simulink model "Tracker_with_Position_Control"  (R2024b)
settings: Solver=FixedStepDiscrete  StartTime=0.0  StopTime=inf  FixedStep=0.005  RelTol=1e-3  EnableMultiTasking=on
libraries: arduinolib x3, simulink x1, arduinosensorlib x1, simulink_extras x1, slpidlib x1
settings Model: ExtModeTrigDuration=2  Creator=yoany  LastModifiedBy=shaha
settings OptimizationCC: DefaultUnderspecifiedDataType=single  EnhancedBackFolding=on  PassReuseOutputArgsThreshold=0  MaxStackSize=64  OptimizeBlockOrder=speed  DifferentSizesBufferReuse=on
settings DebuggingCC: MultiTaskRateTransMsg=warning  ParameterPrecisionLossMsg=none  ParameterTunabilityLossMsg=error
settings HardwareCC: ProdBitPerInt=16  ProdBitPerPointer=16  ProdBitPerSizeT=16  ProdBitPerPtrDiffT=16  ProdLargestAtomicFloat=None  ProdWordSize=8  ProdHWDeviceType=Atmel->AVR  UseEmbeddedCoderFeatures=off
settings SFSimCC: MATLABDynamicMemAlloc=off
settings RTWCC: Description=Embedded Coder  SystemTargetFile=ert.tlc  HardwareBoard=Arduino Uno  TemplateMakefile=ert_default_tmf  Toolchain=Arduino AVR  BuildConfiguration=Faster Runs  GPUComputeCapability=3.5
settings CodeAppCC: ForceParamTrailComments=on  OperatorAnnotations=on
settings ERTTargetCC: ERTCustomFileBanners=off  SupportContinuousTime=on  SupportNonInlinedSFcns=on  RemoveResetFunc=off  SupportVariableSizeSignals=on  ModelStepFunctionPrototypeControlCompliant=off  ExtModeTransport=3  ExtModeStaticAlloc=on  ExtModeAutomaticAllocSize=off  ExtModeStaticAllocSize=250  ExtModeMexFile=ext_xcp  ExtModeIntrfLevel=Level2 - Open  InlinedParameterPlacement=Hierarchical  DynamicArrayContainerType=coder::array

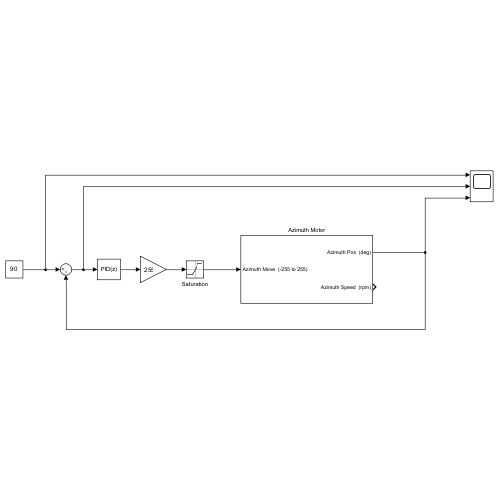
[thumbnail: Simulink's stored preview of the top-level diagram]
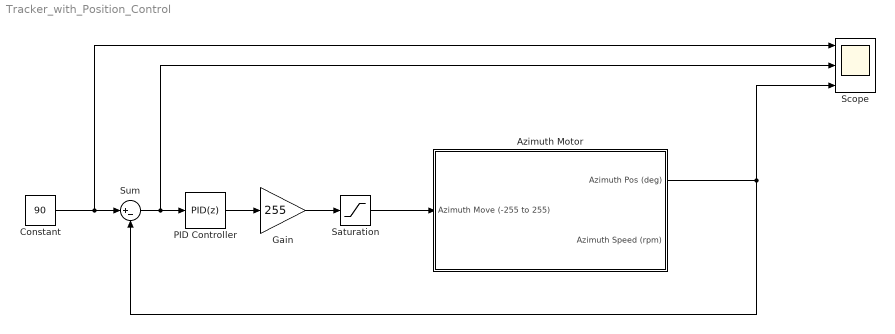
== system Tracker_with_Position_Control ==
  Azimuth Motor : Subsystem
  Constant : Constant  Value=90
  Gain : Gain  Gain=255
  PID Controller : slpidlib/PID Controller  Controller=PID  Form=Parallel  TimeDomain=Discrete-time  UseExternalTs=off  SampleTime=0.01  IntegratorMethod=Forward Euler  FilterMethod=Forward Euler  ControllerParametersSource=internal  P=0.01  I=0.001  UseKiTs=off  D=0  UseExternalDerivativeSource=off  N=100  UseFilter=on  TunerSelectOption=Transfer Function Based (PID Tuner App)  InitialConditionSource=internal  InitialConditionForIntegrator=0  InitialConditionForFilter=0  DifferentiatorICPrevScaledInput=0  ExternalReset=none  TrackingMode=off  Kt=1  LimitOutput=off  SatLimitsSource=internal  UpperSaturationLimit=255  LowerSaturationLimit=-255  LinearizeAsGain=on  AntiWindupMode=none  Kb=1  LimitIntegrator=off  UpperIntegratorSaturationLimit=inf  LowerIntegratorSaturationLimit=-inf  POutMin=[]  POutMax=[]  IOutMin=[]  IOutMax=[]  DOutMin=[]  DOutMax=[]  NOutMin=[]  NOutMax=[]  SumOutMin=[]  SumOutMax=[]  SaturationOutMin=[]  SaturationOutMax=[]  PParamMin=[]  PParamMax=[]  IParamMin=[]  IParamMax=[]  DParamMin=[]  DParamMax=[]  NParamMin=[]  NParamMax=[]  KbParamMin=[]  KbParamMax=[]  KtParamMin=[]  KtParamMax=[]  KbOutMin=[]  KbOutMax=[]  KtOutMin=[]  KtOutMax=[]  IntegratorOutMin=[]  IntegratorOutMax=[]  FilterOutMin=[]  FilterOutMax=[]  SumI1OutMin=[]  SumI1OutMax=[]  SumI2OutMin=[]  SumI2OutMax=[]  SumI3OutMin=[]  SumI3OutMax=[]  SumI4OutMin=[]  SumI4OutMax=[]  SumDOutMin=[]  SumDOutMax=[]  DifferentiatorOutMin=[]  DifferentiatorOutMax=[]  FilterDiffOutCoefMin=[]  FilterDiffOutCoefMax=[]  ReciprocalOutMin=[]  ReciprocalOutMax=[]  SumDenOutMin=[]  SumDenOutMax=[]  SumNumOutMin=[]  SumNumOutMax=[]  DivideOutMin=[]  DivideOutMax=[]  UdiffTsProdOutMin=[]  UdiffTsProdOutMax=[]  NTsProdOutMin=[]  NTsProdOutMax=[]  UintegralTsProdOutMin=[]  UintegralTsProdOutMax=[]  UngainTsProdOutMin=[]  UngainTsProdOutMax=[]  ClampingZeroOutDataTypeStr=Inherit: Inherit via back propagation  ClampingZeroOutMin=[]  ClampingZeroOutMax=[]  FilterDenConstantOutDataTypeStr=Inherit: Inherit via back propagation  FilterDenConstantOutMin=[]  FilterDenConstantOutMax=[]  PCopyOutDataTypeStr=Inherit: Inherit via back propagation  PCopyOutMin=[]  PCopyOutMax=[]  NCopyOutDataTypeStr=Inherit: Inherit via back propagation  NCopyOutMin=[]  NCopyOutMax=[]  IntegratorContinuousStateAttributes=''  IntegratorStateMustResolveToSignalObject=off  IntegratorRTWStateStorageClass=Auto  FilterContinuousStateAttributes=''  FilterStateMustResolveToSignalObject=off  FilterRTWStateStorageClass=Auto  ParallelPVariant=InternalParameters  IdealPVariant=Disabled  IVariant=InternalParameters  DVariant=InternalParameters  IntegratorVariant=Discrete  SatVariant=Disabled  AWVariant=Passthrough  PCopyVariant=Disabled  TRVariant=Disabled  FdbkBlocksVariant=Forward  IdealPFdbkVariant=Disabled  SatFdbkVariant=Disabled  DerivativeFilterVariant=ForwardEulerFilter  NVariant=InternalParameters  NCopyVariant=Disabled  FilterICVariant=InternalICsFilter  IntegratorICVariant=InternalICs  ExternalResetVariant=Disabled  TRSumVariant=Passthrough  SumFdbkVariant=Disabled  SumVariant=Sum_PID  TsampFilterVariant=InternalTs  TsampNgainVariant=Passthrough  TsampIntegralVariant=Disabled_SignalSpec  ExternalSaturationOutDataTypeStr=Inherit: Same as second input  DerivativeSourceVariant=ErrorSignal  PreIntVariant=InternalPreInt
  Saturation : Saturate  UpperLimit=255  LowerLimit=-255
  Scope : Scope  NumInputPorts=3
  Sum : Sum  Inputs=|+-
  wires:
  Constant/1 -> Scope/1, Sum/1
  Sum/1 -> Scope/2, PID Controller/1
  Azimuth Motor/1(Azimuth Pos (deg)) -> Scope/3, Sum/2
  Saturation/1 -> Azimuth Motor/1(Azimuth Move (-255 to 255))
  Gain/1 -> Saturation/1
  PID Controller/1 -> Gain/1

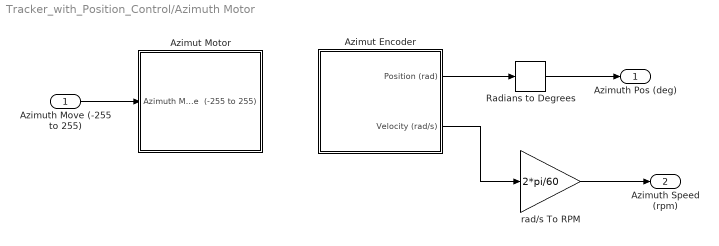
== system Tracker_with_Position_Control/Azimuth Motor ==
  Azimuth Move (-255 to 255) : Inport
  Azimut Encoder : Subsystem
  Azimut Motor : Subsystem
  Radians to Degrees : simulink_extras/Transformations/Radians to Degrees
  rad/s To RPM : Gain  Gain=2*pi/60
  Azimuth Pos (deg) : Outport
  Azimuth Speed (rpm) : Outport  Port=2
  wires:
  Azimut Encoder/2(Velocity (rad/s)) -> rad/s To RPM/1
  Azimut Encoder/1(Position (rad)) -> Radians to Degrees/1
  Azimuth Move (-255 to 255)/1 -> Azimut Motor/1(Azimuth Move  (-255 to 255))
  Radians to Degrees/1 -> Azimuth Pos (deg)/1
  rad/s To RPM/1 -> Azimuth Speed (rpm)/1

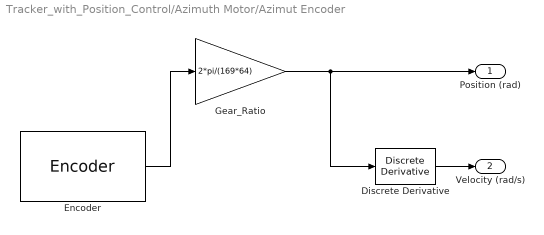
== system Tracker_with_Position_Control/Azimuth Motor/Azimut Encoder ==
  Discrete Derivative : simulink/Quick Insert/Discrete/Discrete Derivative  gainval=1.0  ICPrevScaledInput=0.05  OutMin=[]  OutMax=[]  OutDataType=fixdt(1, 16)  OutScaling=2^-10  DoSatur=off
  Encoder : arduinosensorlib/Encoder  InputA=2  InputB=3  Mode=No reset  SampleTime=0.01
  Gear_Ratio : Gain  Gain=2*pi/(169*64)
  Position (rad) : Outport
  Velocity (rad/s) : Outport  Port=2
  wires:
  Encoder/1 -> Gear_Ratio/1
  Gear_Ratio/1 -> Discrete Derivative/1, Position (rad)/1
  Discrete Derivative/1 -> Velocity (rad/s)/1

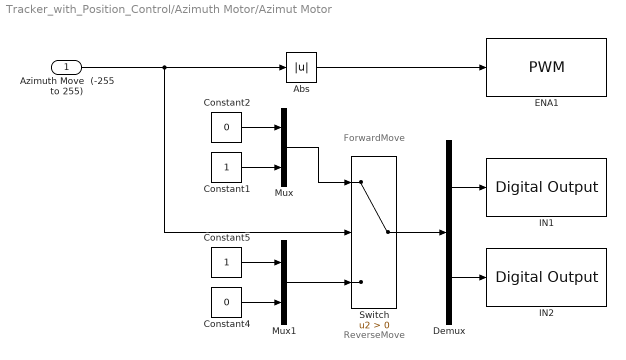
== system Tracker_with_Position_Control/Azimuth Motor/Azimut Motor ==
  note: ForwardMove
  note: ReverseMove
  Azimuth Move  (-255 to 255) : Inport
  Abs : Abs  SaturateOnIntegerOverflow=off
  Constant1 : Constant
  Constant2 : Constant  Value=0
  Constant4 : Constant  Value=0
  Constant5 : Constant
  Demux : Demux  Outputs=2
  ENA1 : arduinolib/PWM  pinNumber=6  frequencyType=Default  desiredFrequency=490.2  achievableFrequency=490.2
  IN1 : arduinolib/Digital Output  pinNumber=7  Direction=output  blockPlatform=arduino
  IN2 : arduinolib/Digital Output  pinNumber=8  Direction=output  blockPlatform=arduino
  Mux : Mux  Inputs=2
  Mux1 : Mux  Inputs=2
  Switch : Switch  Criteria=u2 > Threshold  SaturateOnIntegerOverflow=off  InputSameDT=off
  wires:
  Constant5/1 -> Mux1/1
  Mux/1 -> Switch/1
  Azimuth Move  (-255 to 255)/1 -> Switch/2, Abs/1
  Demux/1 -> IN1/1
  Constant1/1 -> Mux/2
  Constant4/1 -> Mux1/2
  Switch/1 -> Demux/1
  Abs/1 -> ENA1/1
  Demux/2 -> IN2/1
  Mux1/1 -> Switch/3
  Constant2/1 -> Mux/1
